simulink model "gm_hdl_model_fixed"  (R2024a)
settings: Solver=FixedStepDiscrete  StartTime=0.0  StopTime=SIM_TIME  RelTol=1e-3
undefined symbols (not defined in the file or in its folder): a, b, BUFFER_LEN, c, SAMPLING_FREQ, signal_1
libraries: hdlsllib x39, dspsigops x15, simulink_extras x4, simulink x2, dspsrcs4 x1, dsphdlxfrm2 x1
(part 1 of 3)
settings Model: SimulationMode=accelerator  Creator=Jan Rosa  LastModifiedBy=Jan Rosa
settings OptimizationCC: BlockReduction=off  ConditionallyExecuteInputs=off  DefaultParameterBehavior=Inlined  InheritOutputTypeSmallerThanSingle=on
settings DebuggingCC: SignalRangeChecking=warning  AlgebraicLoopMsg=error  SolverPrmCheckMsg=warning  InheritedTsInSrcMsg=none  SingleTaskRateTransMsg=error  UnderSpecifiedDataTypeMsg=warning  UnconnectedInputMsg=error  UnconnectedOutputMsg=error  UnconnectedLineMsg=error  ModelReferenceVersionMismatchMessage=warning  ModelReferenceIOMismatchMessage=warning  ModelReferenceNoExplicitFinalValueMsg=warning  StateNameClashWarn=warning
settings HardwareCC: ProdBitPerPointer=32  ProdBitPerSizeT=32  ProdBitPerPtrDiffT=32  ProdLargestAtomicFloat=None  ProdIntDivRoundTo=Undefined  ProdEndianess=Unspecified  ProdWordSize=32  ProdHWDeviceType=ASIC/FPGA->ASIC/FPGA  TargetBitPerPointer=64  TargetBitPerSizeT=64  TargetBitPerPtrDiffT=64  TargetLongLongMode=on  TargetIntDivRoundTo=Zero  TargetEndianess=LittleEndian  TargetWordSize=64  TargetHWDeviceType=Custom Processor->MATLAB Host Computer  ProdEqTarget=off
settings ModelReferenceCC: EnableRefExpFcnMdlSchedulingChecks=on  EnableParallelModelReferenceBuilds=on

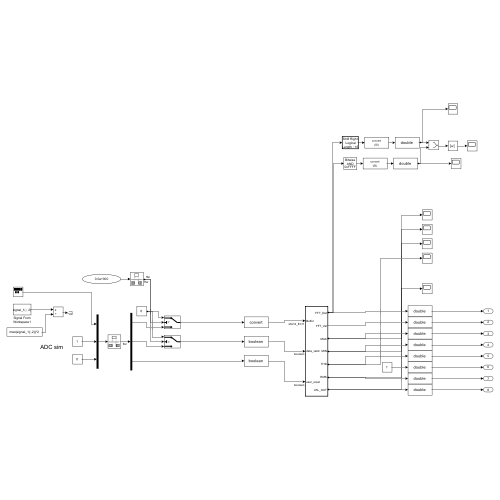
[thumbnail: Simulink's stored preview of the top-level diagram]
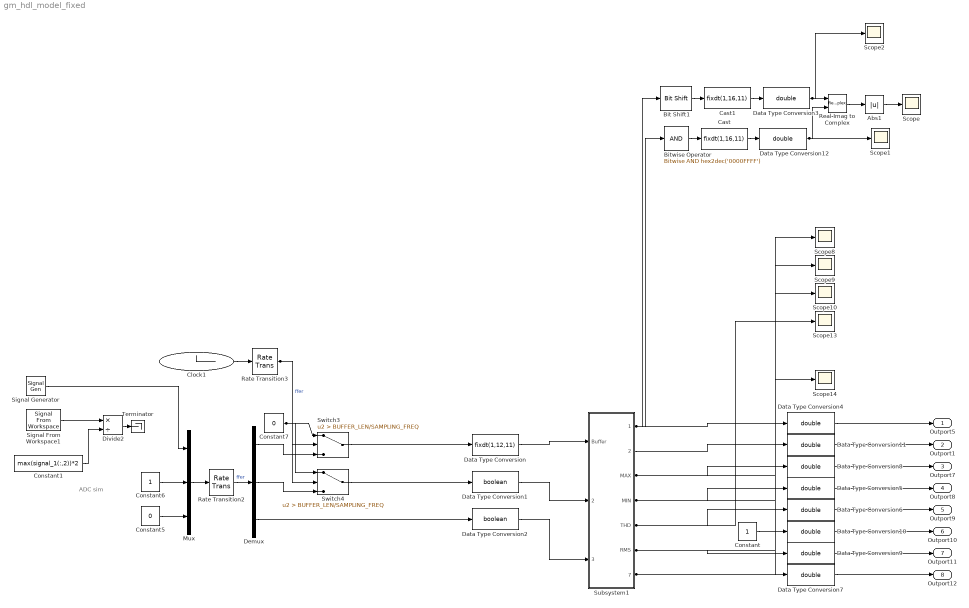
== system gm_hdl_model_fixed ==
  note: ADC sim
  Abs1 : Abs  SaturateOnIntegerOverflow=off
  Bit Shift1 : hdlsllib/Logic and Bit Operations/Bit Shift  mode=Shift Right Logical  N=16
  Bitwise Operator : simulink/Logic and Bit Operations/Bitwise Operator  logicop=AND  UseBitMask=on  BitMask=hex2dec('0000FFFF')  BitMaskRealWorld=Stored Integer
  Cast : DataTypeConversion  OutDataTypeStr=fixdt(1,16,11)  ConvertRealWorld=Stored Integer (SI)  SaturateOnIntegerOverflow=off  RndMeth=Floor
  Cast1 : DataTypeConversion  OutDataTypeStr=fixdt(1,16,11)  ConvertRealWorld=Stored Integer (SI)  SaturateOnIntegerOverflow=off  RndMeth=Floor
  Clock1 : Clock
  Constant : Constant
  Constant1 : Constant  Value=max(signal_1(:,2))*2
  Constant5 : Constant  Value=0
  Constant6 : Constant
  Constant7 : Constant  Value=0  SampleTime=1/SAMPLING_FREQ
  Data Type Conversion : DataTypeConversion  OutDataTypeStr=fixdt(1,12,11)  SaturateOnIntegerOverflow=off  RndMeth=Floor  LockScale=on
  Data Type Conversion1 : DataTypeConversion  OutDataTypeStr=boolean  SaturateOnIntegerOverflow=off  RndMeth=Floor  LockScale=on
  Data Type Conversion{3..12} (10 alike) : DataTypeConversion  OutDataTypeStr=double  SaturateOnIntegerOverflow=off  RndMeth=Floor
  Data Type Conversion2 : DataTypeConversion  OutDataTypeStr=boolean  SaturateOnIntegerOverflow=off  RndMeth=Floor  LockScale=on
  Demux : Demux  Outputs=3
  Divide2 : Product  Inputs=*/
  Mux : Mux  Inputs=3
  Rate Transition2 : RateTransition  Integrity=off  Deterministic=off  OutPortSampleTime=1/SAMPLING_FREQ
  Rate Transition3 : RateTransition  Integrity=off  Deterministic=off  OutPortSampleTime=1/SAMPLING_FREQ
  Real-Imag to Complex : RealImagToComplex
  Scope{,1..2,8..10,13..14} (8 alike) : Scope
  Signal Generator : SignalGenerator  WaveForm=square  Amplitude=0.49999  Frequency=SAMPLING_FREQ/(16*16)
  Signal From Workspace1 : dspsrcs4/Signal From Workspace  X=signal_1(:, 2)  Ts=signal_1(2, 1)  nsamps=1  OutputAfterFinalValue=Cyclic repetition  ignoreOrWarnInputAndFrameLengths=off  OutputFrames=off
  Subsystem1 : Subsystem  TreatAsAtomicUnit=on
  Switch3 : Switch  Criteria=u2 > Threshold  Threshold=BUFFER_LEN/SAMPLING_FREQ  SaturateOnIntegerOverflow=off  InputSameDT=off
  Switch4 : Switch  Criteria=u2 > Threshold  Threshold=BUFFER_LEN/SAMPLING_FREQ  SaturateOnIntegerOverflow=off  InputSameDT=off
  Terminator : Terminator
  Outport5 : Outport
  Outport1 : Outport  Port=2
  Outport7 : Outport  Port=3
  Outport8 : Outport  Port=4
  Outport9 : Outport  Port=5
  Outport10 : Outport  Port=6
  Outport11 : Outport  Port=7
  Outport12 : Outport  Port=8
  wires:
  Divide2/1 -> Terminator/1
  Constant/1 -> Data Type Conversion10/1
  Cast1/1 -> Data Type Conversion3/1
  Cast/1 -> Data Type Conversion12/1
  Data Type Conversion12/1 -> Real-Imag to Complex/2, Scope1/1
  Bitwise Operator/1 -> Cast/1
  Bit Shift1/1 -> Cast1/1
  Signal Generator/1 -> Mux/1
  Real-Imag to Complex/1 -> Abs1/1
  Subsystem1/2(FFT_Val) -> Data Type Conversion11/1
  Data Type Conversion3/1 -> Real-Imag to Complex/1, Scope2/1
  Data Type Conversion11/1 -> Outport1/1
  Data Type Conversion9/1 -> Outport11/1
  Data Type Conversion7/1 -> Outport12/1
  Data Type Conversion10/1 -> Outport10/1
  Data Type Conversion6/1 -> Outport9/1
  Data Type Conversion5/1 -> Outport8/1
  Data Type Conversion8/1 -> Outport7/1
  Data Type Conversion4/1 -> Outport5/1
  Data Type Conversion1/1 -> Subsystem1/2(data_valid)
  Data Type Conversion2/1 -> Subsystem1/3(user_reset)
  Data Type Conversion/1 -> Subsystem1/1(Buffer)
  Subsystem1/6(RMS) -> Scope8/1, Data Type Conversion9/1
  Constant1/1 -> Divide2/2
  Constant6/1 -> Mux/2
  Signal From Workspace1/1 -> Divide2/1
  Constant5/1 -> Mux/3
  Rate Transition2/1 -> Demux/1  "ffer"
  Abs1/1 -> Scope/1
  Subsystem1/4(MIN) -> Scope9/1, Data Type Conversion5/1
  Mux/1 -> Rate Transition2/1
  Demux/1 -> Switch3/3
  Switch3/1 -> Data Type Conversion/1
  Subsystem1/5(THD) -> Scope13/1, Data Type Conversion6/1
  Demux/3 -> Data Type Conversion2/1
  Clock1/1 -> Rate Transition3/1
  Demux/2 -> Switch4/3
  Subsystem1/3(MAX) -> Scope10/1, Data Type Conversion8/1
  Subsystem1/7(VAL_OUT) -> Scope14/1, Data Type Conversion7/1
  Rate Transition3/1 -> Switch3/2, Switch4/2  "ffer"
  Constant7/1 -> Switch3/1, Switch4/1
  Switch4/1 -> Data Type Conversion1/1
  Subsystem1/1(FFT_Dat) -> Bit Shift1/1, Bitwise Operator/1, Data Type Conversion4/1

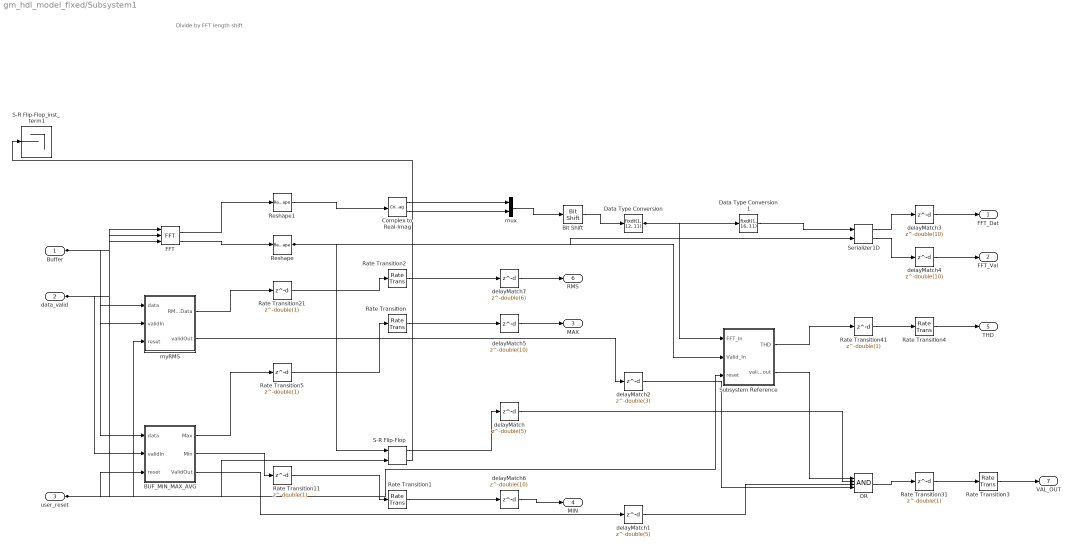
== system gm_hdl_model_fixed/Subsystem1 ==
  note: Divide by FFT length shift
  Buffer : Inport  OutDataTypeStr=fixdt(1, 12, 11)  PortDimensions=1  SampleTime=1e-08
  data_valid : Inport  Port=2  OutDataTypeStr=boolean  PortDimensions=1  SampleTime=1e-08
  user_reset : Inport  Port=3  OutDataTypeStr=boolean  PortDimensions=1  SampleTime=1e-08
  BUF_MIN_MAX_AVG : Subsystem
  Bit Shift : hdlsllib/Logic and Bit Operations/Bit Shift  mode=Shift Right Arithmetic  N=double(11)
  Complex to Real-Imag : ComplexToRealImag  SampleTime=1e-08
  Data Type Conversion : DataTypeConversion  OutDataTypeStr=fixdt(1, 12, 11)  SampleTime=1e-08  SaturateOnIntegerOverflow=off  RndMeth=Floor
  Data Type Conversion1 : DataTypeConversion  OutDataTypeStr=fixdt(1, 16, 11)  SampleTime=1e-08  SaturateOnIntegerOverflow=off  RndMeth=Floor
  FFT : dsphdlxfrm2/FFT  Architecture=Streaming Radix 2^2  FFTLengthSource=Property  FFTLength=BUFFER_LEN  FFTLengthMax=1024  ComplexMultiplication=Use 4 multipliers and 2 adders  BitReversedOutput=off  BitReversedInput=off  Normalize=off  SimulateUsing=Code generation  RoundingMethod=Floor  ResetInputPort=on  StartOutputPort=off  EndOutputPort=off
  OR : Logic  Inputs=4  AllPortsSameDT=off  OutDataTypeStr=boolean  SampleTime=1e-08
  Rate Transition : RateTransition  Integrity=off  Deterministic=off  InitialCondition="fi(0,0,16,16,\"hex\",\"0000\")"  OutPortSampleTimeOpt=Multiple of input port sample time  OutPortSampleTimeMultiple=1/2
  Rate Transition1 : RateTransition  Integrity=off  Deterministic=off  InitialCondition="fi(0,1,16,15,\"hex\",\"0000\")"  OutPortSampleTimeOpt=Multiple of input port sample time  OutPortSampleTimeMultiple=1/2
  Rate Transition{5,11,21,31,41} (5 alike) : Delay  DelayLength=double(1)  InitialCondition=0  SampleTime=1e-08
  Rate Transition2 : RateTransition  Integrity=off  Deterministic=off  InitialCondition="fi(0,0,16,7,\"hex\",\"0000\")"  OutPortSampleTimeOpt=Multiple of input port sample time  OutPortSampleTimeMultiple=1/2
  Rate Transition3 : RateTransition  Integrity=off  Deterministic=off  OutPortSampleTimeOpt=Multiple of input port sample time  OutPortSampleTimeMultiple=1/2
  Rate Transition4 : RateTransition  Integrity=off  Deterministic=off  InitialCondition="fi(0,1,18,10,\"hex\",\"00000\")"  OutPortSampleTimeOpt=Multiple of input port sample time  OutPortSampleTimeMultiple=1/2
  Reshape : Reshape
  Reshape1 : Reshape
  S-R Flip-Flop : simulink_extras/Flip Flops/S-R Flip-Flop  initial_condition=0
  S-R Flip-Flop_inst_term1 : Terminator
  Serializer1D : hdlsllib/HDL Operations/Serializer1D  Ratio=2  IdleCycles=0  validIn=on  startOut=off  validOut=on  inputDataDimensions=2  inputSampleTime=1e-08  inputSignalType=real
  Subsystem Reference : Subsystem
  delayMatch : Delay  DelayLength=double(5)  InitialCondition=0  SampleTime=1e-08
  delayMatch1 : Delay  DelayLength=double(5)  InitialCondition=0  SampleTime=1e-08
  delayMatch2 : Delay  DelayLength=double(3)  InitialCondition=0  SampleTime=1e-08
  delayMatch{3..6} (4 alike) : Delay  DelayLength=double(10)  InitialCondition=0  SampleTime=5e-09
  delayMatch7 : Delay  DelayLength=double(6)  InitialCondition=0  SampleTime=5e-09
  mux : Mux  Inputs=2
  myRMS : Subsystem
  FFT_Dat : Outport  SampleTime=5e-09
  FFT_Val : Outport  Port=2  SampleTime=5e-09
  MAX : Outport  Port=3  SampleTime=5e-09
  MIN : Outport  Port=4  SampleTime=5e-09
  THD : Outport  Port=5  SampleTime=5e-09
  RMS : Outport  Port=6  SampleTime=5e-09
  VAL_OUT : Outport  Port=7  SampleTime=5e-09
  wires:
  Buffer/1 -> BUF_MIN_MAX_AVG/1(data), myRMS/1(data), FFT/1
  data_valid/1 -> BUF_MIN_MAX_AVG/2(validIn), myRMS/2(validIn), FFT/2
  user_reset/1 -> myRMS/3(reset), BUF_MIN_MAX_AVG/3(reset), Subsystem Reference/3(reset), S-R Flip-Flop/2, FFT/3
  BUF_MIN_MAX_AVG/1(Max) -> Rate Transition5/1
  BUF_MIN_MAX_AVG/2(Min) -> Rate Transition11/1
  delayMatch1/1 -> OR/3
  Data Type Conversion/1 -> Subsystem Reference/1(FFT_In), Data Type Conversion1/1
  FFT/1 -> Reshape1/1
  FFT/2 -> Reshape/1
  Reshape/1 -> Subsystem Reference/2(Valid_In), Serializer1D/2, S-R Flip-Flop/1
  delayMatch3/1 -> FFT_Dat/1
  Subsystem Reference/1(THD) -> Rate Transition41/1
  Subsystem Reference/2(valid_out) -> OR/1
  myRMS/1(RMS_Data) -> Rate Transition21/1
  delayMatch2/1 -> OR/4
  delayMatch5/1 -> MAX/1
  delayMatch6/1 -> MIN/1
  delayMatch7/1 -> RMS/1
  Rate Transition3/1 -> VAL_OUT/1
  Rate Transition4/1 -> THD/1
  delayMatch4/1 -> FFT_Val/1
  delayMatch/1 -> OR/2
  Rate Transition5/1 -> Rate Transition/1
  Rate Transition11/1 -> Rate Transition1/1
  Rate Transition21/1 -> Rate Transition2/1
  Rate Transition31/1 -> Rate Transition3/1
  Rate Transition41/1 -> Rate Transition4/1
  S-R Flip-Flop/2 -> S-R Flip-Flop_inst_term1/1
  Reshape1/1 -> Complex to Real-Imag/1
  Complex to Real-Imag/1 -> mux/1
  Complex to Real-Imag/2 -> mux/2
  mux/1 -> Bit Shift/1
  Bit Shift/1 -> Data Type Conversion/1
  Data Type Conversion1/1 -> Serializer1D/1
  OR/1 -> Rate Transition31/1
  S-R Flip-Flop/1 -> delayMatch/1
  BUF_MIN_MAX_AVG/3(ValidOut) -> delayMatch1/1
  myRMS/2(validOut) -> delayMatch2/1
  Serializer1D/1 -> delayMatch3/1
  Serializer1D/2 -> delayMatch4/1
  Rate Transition/1 -> delayMatch5/1
  Rate Transition1/1 -> delayMatch6/1
  Rate Transition2/1 -> delayMatch7/1

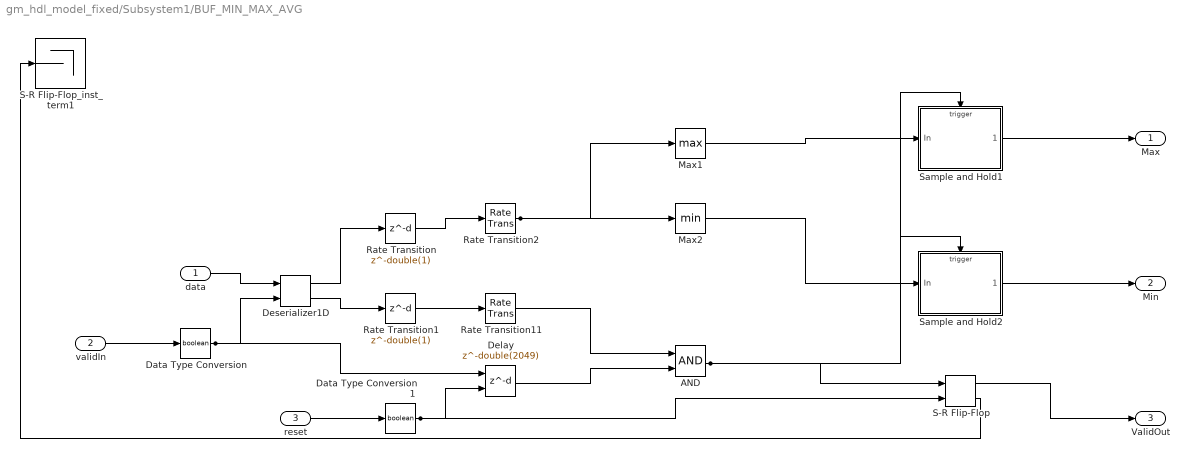
== system gm_hdl_model_fixed/Subsystem1/BUF_MIN_MAX_AVG ==
  data : Inport  OutDataTypeStr=fixdt(1, 12, 11)  PortDimensions=1  SampleTime=1e-08
  validIn : Inport  Port=2  OutDataTypeStr=boolean  PortDimensions=1  SampleTime=1e-08
  reset : Inport  Port=3  OutDataTypeStr=boolean  PortDimensions=1  SampleTime=1e-08
  AND : Logic  AllPortsSameDT=off  OutDataTypeStr=boolean  SampleTime=1e-08
  Data Type Conversion : DataTypeConversion  OutDataTypeStr=boolean
  Data Type Conversion1 : DataTypeConversion  OutDataTypeStr=boolean
  Delay : Delay  DelayLength=double(2049)  InitialCondition=0  ExternalReset=Level
      settings: InputPortMap=u0,r5
  Deserializer1D : hdlsllib/HDL Operations/Deserializer1D  Ratio=2048  IdleCycles=0  InitialCondition=0  startIn=off  validIn=on  validOut=on  inputDataDimensions=1  inputSampleTime=1e-08  inputSignalType=real
  Max1 : MinMax  Function=max  OutDataTypeStr=fixdt(0,16,16)
  Max2 : MinMax  OutDataTypeStr=fixdt(1,16,15)
  Rate Transition : Delay  DelayLength=double(1)  InitialCondition=0  SampleTime=2.048e-05
  Rate Transition1 : Delay  DelayLength=double(1)  InitialCondition=0  SampleTime=2.048e-05
  Rate Transition11 : RateTransition  Integrity=off  Deterministic=off  OutPortSampleTimeOpt=Multiple of input port sample time  OutPortSampleTimeMultiple=1/2048
  Rate Transition2 : RateTransition  Integrity=off  Deterministic=off  InitialCondition="fi(0,1,12,11,\"hex\",\"000\")"  OutPortSampleTimeOpt=Multiple of input port sample time  OutPortSampleTimeMultiple=1/2048
  S-R Flip-Flop : simulink_extras/Flip Flops/S-R Flip-Flop  initial_condition=0
  S-R Flip-Flop_inst_term1 : Terminator
  Sample and Hold1 : Subsystem  mask(Sample and Hold){trig=Rising edge, initCond=double(0), latchinput=off}
      mask prompts: trig "dsp:DSPSignalOperationsBlockDialog:TriggerType_MP"; initCond "dsp:DSPSignalOperationsBlockDialog:InitialCondition_MP"; latchinput "dsp:DSPSignalOperationsBlockDialog:LatchInput_MP"
      mask help: dsp:DSPSignalOperationsBlockDialog:SampleAndHold_MaskDesc
      mask init:
      | initCond = double(0);
      | latchinput = double(0);
      | s = 'rising';
      | trig = double(1);
      mask Help: eval('blocksethelp');
      mask TypeOptions trig: dsp:DSPSignalOperationsBlockDialog:RisingEdge_MP | dsp:DSPSignalOperationsBlockDialog:FallingEdge_MP | dsp:DSPSignalOperationsBlockDialog:EitherEdge_MP
      mask Display: disp('S/H')
  Sample and Hold2 : Subsystem  mask(Sample and Hold){trig=Rising edge, initCond=double(0), latchinput=off}
      mask prompts: trig "dsp:DSPSignalOperationsBlockDialog:TriggerType_MP"; initCond "dsp:DSPSignalOperationsBlockDialog:InitialCondition_MP"; latchinput "dsp:DSPSignalOperationsBlockDialog:LatchInput_MP"
      mask help: dsp:DSPSignalOperationsBlockDialog:SampleAndHold_MaskDesc
      mask init:
      | initCond = double(0);
      | latchinput = double(0);
      | s = 'rising';
      | trig = double(1);
      mask Help: eval('blocksethelp');
      mask TypeOptions trig: dsp:DSPSignalOperationsBlockDialog:RisingEdge_MP | dsp:DSPSignalOperationsBlockDialog:FallingEdge_MP | dsp:DSPSignalOperationsBlockDialog:EitherEdge_MP
      mask Display: disp('S/H')
  Max : Outport  SampleTime=1e-08
  Min : Outport  Port=2  SampleTime=1e-08
  ValidOut : Outport  Port=3  SampleTime=1e-08
  wires:
  data/1 -> Deserializer1D/1
  validIn/1 -> Data Type Conversion/1
  reset/1 -> Data Type Conversion1/1
  Delay/1 -> AND/2
  S-R Flip-Flop/1 -> ValidOut/1
  Sample and Hold1/1(" ") -> Max/1
  Sample and Hold2/1(" ") -> Min/1
  Deserializer1D/2 -> Rate Transition1/1
  Data Type Conversion1/1 -> Delay/2, S-R Flip-Flop/2
  Max2/1 -> Sample and Hold2/1(In)
  Max1/1 -> Sample and Hold1/1(In)
  Rate Transition1/1 -> Rate Transition11/1
  Rate Transition/1 -> Rate Transition2/1
  Rate Transition11/1 -> AND/1
  Rate Transition2/1 -> Max2/1, Max1/1
  Data Type Conversion/1 -> Deserializer1D/2, Delay/1
  AND/1 -> Sample and Hold1/Trigger, Sample and Hold2/Trigger, S-R Flip-Flop/1
  S-R Flip-Flop/2 -> S-R Flip-Flop_inst_term1/1
  Deserializer1D/1 -> Rate Transition/1

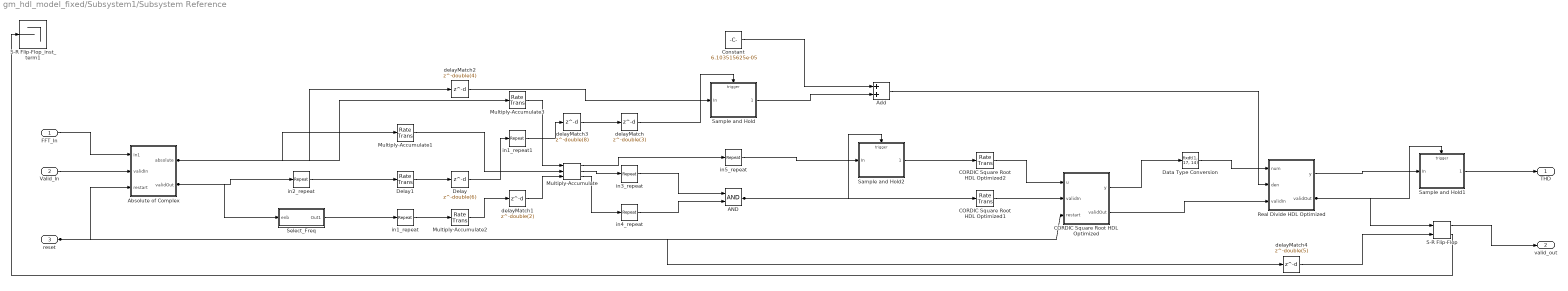
== system gm_hdl_model_fixed/Subsystem1/Subsystem Reference ==
  FFT_In : Inport  OutDataTypeStr=fixdt(1, 12, 11)  PortDimensions=[2]  SampleTime=1e-08
  Valid_In : Inport  Port=2  OutDataTypeStr=boolean  PortDimensions=1  SampleTime=1e-08
  reset : Inport  Port=3  OutDataTypeStr=boolean  PortDimensions=1  SampleTime=1e-08
  AND : Logic  AllPortsSameDT=off  OutDataTypeStr=boolean  SampleTime=5e-09
  Absolute of Complex : Subsystem
  Add : Sum  OutDataTypeStr=fixdt(1, 17, 14)  AccumDataTypeStr=fixdt(1, 17, 14)  SampleTime=5e-09
  CORDIC Square Root HDL Optimized : Subsystem  mask(CORDIC Square Root HDL Optimized){autoMaximumShiftVal=on, maximumShiftValue=double(10), nIterPerReg=double(1)}
      mask prompts: autoMaximumShiftVal "fixed:emblib:AutoCORDICMaxShiftValue"; maximumShiftValue "fixed:emblib:CORDICMaxShiftValue"; nIterPerReg "fixed:emblib:NumberOfIterationsPerReg"
      mask help: fixed:emblib:CORDICSquareRootHDLFullDescription
      mask Help: eval('embblk.embhelp(gcb)')
      mask Callback autoMaximumShiftVal:
      | autoMaxShiftVal = get_param(gcb,'autoMaximumShiftVal');
      | if strcmp(autoMaxShiftVal,'on')
      |     set_param(gcb,'MaskVisibilities',{'on','off','on'});
      | else
      |     set_param(gcb,'MaskVisibilities',{'on','on','on'});
      | end
      mask Display: disp('CORDIC Square Root\nHDL Optimized')
  CORDIC Square Root HDL Optimized1 : RateTransition  OutPortSampleTimeOpt=Multiple of input port sample time  OutPortSampleTimeMultiple=2
  CORDIC Square Root HDL Optimized2 : RateTransition  OutPortSampleTimeOpt=Multiple of input port sample time  OutPortSampleTimeMultiple=2
  Constant : Constant  Value=6.103515625e-05  OutDataTypeStr=fixdt(1, 16, 14)  SampleTime=5e-09
  Data Type Conversion : DataTypeConversion  OutDataTypeStr=fixdt(1, 17, 14)  SampleTime=1e-08  SaturateOnIntegerOverflow=off  RndMeth=Floor
  Delay : Delay  DelayLength=double(6)  InitialCondition=0  SampleTime=1e-08
  Delay1 : RateTransition  OutPortSampleTimeOpt=Multiple of input port sample time  OutPortSampleTimeMultiple=2
  Multiply-Accumulate : hdlsllib/HDL Operations/Multiply-Accumulate  opMode=Streaming - using Number of Samples  initValueSetting=Dialog  initValue=0  initValueSetting2=Dialog  initValue2=0  initValueSetting3=Dialog  initValue3=0  num_samples=1015  RndMeth2=Floor  RndMeth3=Floor  datatype2=Inherit: Inherit via back propagation  datatype3=fixdt(1, 22, 20)  validOut=on  endInandOut=on  startOut=on  countOut=off  dim=-1  DoSatur=off  parallel=off
  Multiply-Accumulate1 : RateTransition  OutPortSampleTimeOpt=Multiple of input port sample time  OutPortSampleTimeMultiple=2
  Multiply-Accumulate2 : RateTransition  OutPortSampleTimeOpt=Multiple of input port sample time  OutPortSampleTimeMultiple=2
  Multiply-Accumulate3 : RateTransition  OutPortSampleTimeOpt=Multiple of input port sample time  OutPortSampleTimeMultiple=2
  Real Divide HDL Optimized : Subsystem  mask(Real Divide HDL Optimized){OutputType=fixdt(1,18,10)}
      mask prompts: OutputType "fixed:emblib:OutputPrototype"
      mask help: fixed:emblib:RealDivideFullDescription
      mask Help: eval('embblk.embhelp(gcb)')
      mask Display:
      | text(0.5,0.6,'den ~= 0','texmode','on','HorizontalAlignment','center')
      | text(0.5,0.4,'y = num/den','texmode','on','HorizontalAlignment','center')
  S-R Flip-Flop : simulink_extras/Flip Flops/S-R Flip-Flop  initial_condition=0
  S-R Flip-Flop_inst_term1 : Terminator
  Sample and Hold : Subsystem  mask(Sample and Hold){trig=Rising edge, initCond=double(0), latchinput=off}
      mask prompts: trig "dsp:DSPSignalOperationsBlockDialog:TriggerType_MP"; initCond "dsp:DSPSignalOperationsBlockDialog:InitialCondition_MP"; latchinput "dsp:DSPSignalOperationsBlockDialog:LatchInput_MP"
      mask help: dsp:DSPSignalOperationsBlockDialog:SampleAndHold_MaskDesc
      mask init:
      | initCond = double(0);
      | latchinput = double(0);
      | s = 'rising';
      | trig = double(1);
      mask Help: eval('blocksethelp');
      mask TypeOptions trig: dsp:DSPSignalOperationsBlockDialog:RisingEdge_MP | dsp:DSPSignalOperationsBlockDialog:FallingEdge_MP | dsp:DSPSignalOperationsBlockDialog:EitherEdge_MP
      mask Display: disp('S/H')
  Sample and Hold1 : Subsystem  mask(Sample and Hold){trig=Rising edge, initCond=double(0), latchinput=off}
      mask prompts: trig "dsp:DSPSignalOperationsBlockDialog:TriggerType_MP"; initCond "dsp:DSPSignalOperationsBlockDialog:InitialCondition_MP"; latchinput "dsp:DSPSignalOperationsBlockDialog:LatchInput_MP"
      mask help: dsp:DSPSignalOperationsBlockDialog:SampleAndHold_MaskDesc
      mask init:
      | initCond = double(0);
      | latchinput = double(0);
      | s = 'rising';
      | trig = double(1);
      mask Help: eval('blocksethelp');
      mask TypeOptions trig: dsp:DSPSignalOperationsBlockDialog:RisingEdge_MP | dsp:DSPSignalOperationsBlockDialog:FallingEdge_MP | dsp:DSPSignalOperationsBlockDialog:EitherEdge_MP
      mask Display: disp('S/H')
  Sample and Hold2 : Subsystem  mask(Sample and Hold){trig=Rising edge, initCond=double(0), latchinput=off}
      mask prompts: trig "dsp:DSPSignalOperationsBlockDialog:TriggerType_MP"; initCond "dsp:DSPSignalOperationsBlockDialog:InitialCondition_MP"; latchinput "dsp:DSPSignalOperationsBlockDialog:LatchInput_MP"
      mask help: dsp:DSPSignalOperationsBlockDialog:SampleAndHold_MaskDesc
      mask init:
      | initCond = double(0);
      | latchinput = double(0);
      | s = 'rising';
      | trig = double(1);
      mask Help: eval('blocksethelp');
      mask TypeOptions trig: dsp:DSPSignalOperationsBlockDialog:RisingEdge_MP | dsp:DSPSignalOperationsBlockDialog:FallingEdge_MP | dsp:DSPSignalOperationsBlockDialog:EitherEdge_MP
      mask Display: disp('S/H')
  Select_Freq : Subsystem
  delayMatch : Delay  DelayLength=double(3)  InitialCondition=0  SampleTime=5e-09
  delayMatch1 : Delay  DelayLength=double(2)  InitialCondition=0  SampleTime=1e-08
  delayMatch2 : Delay  DelayLength=double(4)  InitialCondition=0  SampleTime=5e-09
  delayMatch3 : Delay  DelayLength=double(8)  InitialCondition=0  SampleTime=5e-09
  delayMatch4 : Delay  DelayLength=double(5)  InitialCondition=0  SampleTime=1e-08
  in1_repeat : dspsigops/Repeat  FactorSource=Dialog parameter  N=double(2)  Nmax=16  RateOptions=Allow multirate processing  ic=0  mode=Unused parameter value
  in1_repeat1 : dspsigops/Repeat  FactorSource=Dialog parameter  N=double(2)  Nmax=16  RateOptions=Allow multirate processing  ic=0  mode=Unused parameter value
  in2_repeat : dspsigops/Repeat  FactorSource=Dialog parameter  N=double(2)  Nmax=16  RateOptions=Allow multirate processing  ic=0  mode=Unused parameter value
  in3_repeat : dspsigops/Repeat  FactorSource=Dialog parameter  N=double(2)  Nmax=16  RateOptions=Allow multirate processing  ic=0  mode=Unused parameter value
  in4_repeat : dspsigops/Repeat  FactorSource=Dialog parameter  N=double(2)  Nmax=16  RateOptions=Allow multirate processing  ic=0  mode=Unused parameter value
  in5_repeat : dspsigops/Repeat  FactorSource=Dialog parameter  N=double(2)  Nmax=16  RateOptions=Allow multirate processing  ic=0  mode=Unused parameter value
  THD : Outport  SampleTime=1e-08
  valid_out : Outport  Port=2  SampleTime=1e-08
  wires:
  FFT_In/1 -> Absolute of Complex/1(In1)
  Valid_In/1 -> Absolute of Complex/2(validIn)
  delayMatch4/1 -> S-R Flip-Flop/2
  CORDIC Square Root HDL Optimized1/1 -> CORDIC Square Root HDL Optimized/2(validIn)
  Absolute of Complex/2(validOut) -> Select_Freq/1(enb), in2_repeat/1
  CORDIC Square Root HDL Optimized/1(y) -> Data Type Conversion/1
  CORDIC Square Root HDL Optimized/2(validOut) -> Real Divide HDL Optimized/3(validIn)
  Data Type Conversion/1 -> Real Divide HDL Optimized/1(num)
  Multiply-Accumulate/1 -> in5_repeat/1
  Multiply-Accumulate/2 -> in3_repeat/1
  Multiply-Accumulate/3 -> in4_repeat/1
  Real Divide HDL Optimized/1(y) -> Sample and Hold1/1(In)
  Real Divide HDL Optimized/2(validOut) -> Sample and Hold1/Trigger, S-R Flip-Flop/1
  S-R Flip-Flop/1 -> valid_out/1
  Sample and Hold1/1(" ") -> THD/1
  CORDIC Square Root HDL Optimized2/1 -> CORDIC Square Root HDL Optimized/1(u)
  Select_Freq/1(Out1) -> in1_repeat/1
  S-R Flip-Flop/2 -> S-R Flip-Flop_inst_term1/1
  Add/1 -> Real Divide HDL Optimized/2(den)
  delayMatch2/1 -> Sample and Hold/1(In)
  Delay1/1 -> Delay/1
  Multiply-Accumulate1/1 -> Multiply-Accumulate/2
  delayMatch1/1 -> Multiply-Accumulate/3
  Delay/1 -> in1_repeat1/1
  Multiply-Accumulate3/1 -> Multiply-Accumulate/1
  in1_repeat/1 -> Multiply-Accumulate2/1
  in2_repeat/1 -> Delay1/1
  Constant/1 -> Add/1
  delayMatch3/1 -> delayMatch/1
  in3_repeat/1 -> AND/1
  in4_repeat/1 -> AND/2
  in5_repeat/1 -> Sample and Hold2/1(In)
  AND/1 -> CORDIC Square Root HDL Optimized1/1, Sample and Hold2/Trigger
  Sample and Hold2/1(" ") -> CORDIC Square Root HDL Optimized2/1
  Multiply-Accumulate2/1 -> delayMatch1/1
  Absolute of Complex/1(absolute) -> delayMatch2/1, Multiply-Accumulate3/1, Multiply-Accumulate1/1
  in1_repeat1/1 -> delayMatch3/1
  reset/1 -> delayMatch4/1, Absolute of Complex/3(restart), CORDIC Square Root HDL Optimized/3(restart)
  delayMatch/1 -> Sample and Hold/Trigger
  Sample and Hold/1(" ") -> Add/2

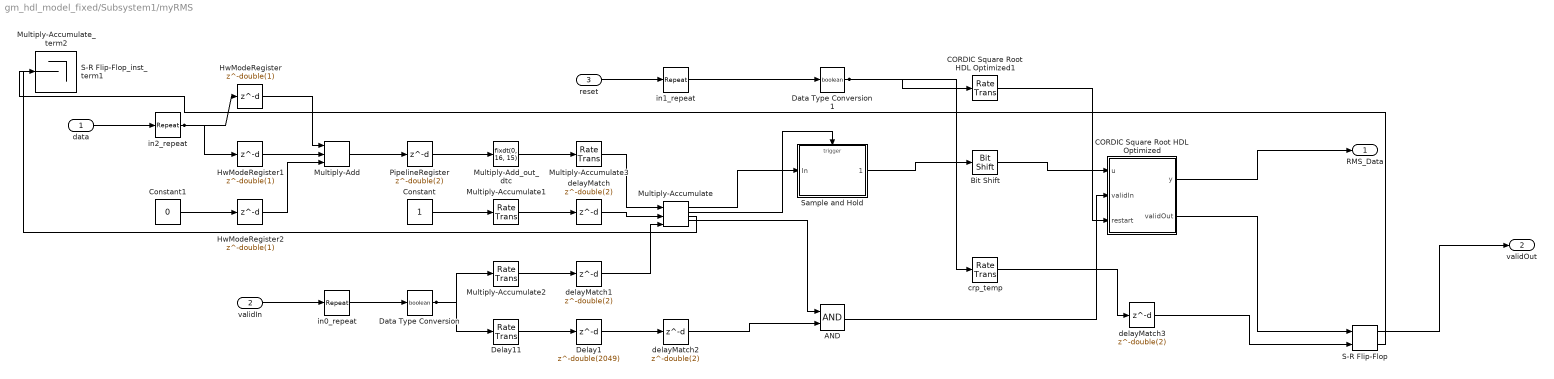
== system gm_hdl_model_fixed/Subsystem1/myRMS ==
  data : Inport  OutDataTypeStr=fixdt(1, 12, 11)  PortDimensions=1  SampleTime=1e-08
  validIn : Inport  Port=2  OutDataTypeStr=boolean  PortDimensions=1  SampleTime=1e-08
  reset : Inport  Port=3  OutDataTypeStr=boolean  PortDimensions=1  SampleTime=1e-08
  AND : Logic  AllPortsSameDT=off  OutDataTypeStr=boolean  SampleTime=1e-08
  Bit Shift : hdlsllib/Logic and Bit Operations/Bit Shift  mode=Shift Right Arithmetic  N=double(11)
  CORDIC Square Root HDL Optimized : Subsystem  mask(CORDIC Square Root HDL Optimized){autoMaximumShiftVal=on, maximumShiftValue=double(10), nIterPerReg=double(1)}
      mask prompts: autoMaximumShiftVal "fixed:emblib:AutoCORDICMaxShiftValue"; maximumShiftValue "fixed:emblib:CORDICMaxShiftValue"; nIterPerReg "fixed:emblib:NumberOfIterationsPerReg"
      mask help: fixed:emblib:CORDICSquareRootHDLFullDescription
      mask Help: eval('embblk.embhelp(gcb)')
      mask Callback autoMaximumShiftVal:
      | autoMaxShiftVal = get_param(gcb,'autoMaximumShiftVal');
      | if strcmp(autoMaxShiftVal,'on')
      |     set_param(gcb,'MaskVisibilities',{'on','off','on'});
      | else
      |     set_param(gcb,'MaskVisibilities',{'on','on','on'});
      | end
      mask Display: disp('CORDIC Square Root\nHDL Optimized')
  CORDIC Square Root HDL Optimized1 : RateTransition  OutPortSampleTimeOpt=Multiple of input port sample time  OutPortSampleTimeMultiple=2
  Constant : Constant  OutDataTypeStr=fixdt(0, 16, 15)  SampleTime=5e-09
  Constant1 : Constant  Value=0  OutDataTypeStr=fixdt(1, 12, 11)  SampleTime=5e-09
  Data Type Conversion : DataTypeConversion  OutDataTypeStr=boolean
  Data Type Conversion1 : DataTypeConversion  OutDataTypeStr=boolean
  Delay1 : Delay  DelayLength=double(2049)  InitialCondition=0  SampleTime=1e-08
  Delay11 : RateTransition  OutPortSampleTimeOpt=Multiple of input port sample time  OutPortSampleTimeMultiple=2
  HwModeRegister : Delay  DelayLength=double(1)  InitialCondition=0  SampleTime=5e-09
  HwModeRegister1 : Delay  DelayLength=double(1)  InitialCondition=0  SampleTime=5e-09
  HwModeRegister2 : Delay  DelayLength=double(1)  InitialCondition=0  SampleTime=5e-09
  Multiply-Accumulate : hdlsllib/HDL Operations/Multiply-Accumulate  opMode=Streaming - using Number of Samples  initValueSetting=Dialog  initValue=0  initValueSetting2=Dialog  initValue2=0  initValueSetting3=Dialog  initValue3=0  num_samples=2048  RndMeth2=Floor  RndMeth3=Floor  datatype2=Inherit: Inherit via back propagation  datatype3=fixdt(0, 16, 7)  validOut=on  endInandOut=on  startOut=on  countOut=on  dim=-1  DoSatur=off  parallel=off
  Multiply-Accumulate1 : RateTransition  OutPortSampleTimeOpt=Multiple of input port sample time  OutPortSampleTimeMultiple=2
  Multiply-Accumulate2 : RateTransition  OutPortSampleTimeOpt=Multiple of input port sample time  OutPortSampleTimeMultiple=2
  Multiply-Accumulate3 : RateTransition  OutPortSampleTimeOpt=Multiple of input port sample time  OutPortSampleTimeMultiple=2
  Multiply-Accumulate_term2 : Terminator
  Multiply-Add : hdlsllib/HDL Operations/Multiply-Add  Function=c+(a.*b)  datatype=fixdt(1, 25, 22)  DoSatur=off  FMA=off
  Multiply-Add_out_dtc : DataTypeConversion  OutDataTypeStr=fixdt(0, 16, 15)  SampleTime=5e-09  SaturateOnIntegerOverflow=off  RndMeth=Floor
  PipelineRegister : Delay  DelayLength=double(2)  InitialCondition=0  SampleTime=5e-09
  S-R Flip-Flop : simulink_extras/Flip Flops/S-R Flip-Flop  initial_condition=0
  S-R Flip-Flop_inst_term1 : Terminator
  Sample and Hold : Subsystem  mask(Sample and Hold){trig=Rising edge, initCond=double(0), latchinput=off}
      mask prompts: trig "dsp:DSPSignalOperationsBlockDialog:TriggerType_MP"; initCond "dsp:DSPSignalOperationsBlockDialog:InitialCondition_MP"; latchinput "dsp:DSPSignalOperationsBlockDialog:LatchInput_MP"
      mask help: dsp:DSPSignalOperationsBlockDialog:SampleAndHold_MaskDesc
      mask init:
      | initCond = double(0);
      | latchinput = double(0);
      | s = 'rising';
      | trig = double(1);
      mask Help: eval('blocksethelp');
      mask TypeOptions trig: dsp:DSPSignalOperationsBlockDialog:RisingEdge_MP | dsp:DSPSignalOperationsBlockDialog:FallingEdge_MP | dsp:DSPSignalOperationsBlockDialog:EitherEdge_MP
      mask Display: disp('S/H')
  crp_temp : RateTransition  OutPortSampleTimeOpt=Multiple of input port sample time  OutPortSampleTimeMultiple=2
  delayMatch{,1..3} (4 alike) : Delay  DelayLength=double(2)  InitialCondition=0  SampleTime=1e-08
  in0_repeat : dspsigops/Repeat  FactorSource=Dialog parameter  N=double(2)  Nmax=16  RateOptions=Allow multirate processing  ic=0  mode=Unused parameter value
  in1_repeat : dspsigops/Repeat  FactorSource=Dialog parameter  N=double(2)  Nmax=16  RateOptions=Allow multirate processing  ic=0  mode=Unused parameter value
  in2_repeat : dspsigops/Repeat  FactorSource=Dialog parameter  N=double(2)  Nmax=16  RateOptions=Allow multirate processing  ic=0  mode=Unused parameter value
  RMS_Data : Outport  SampleTime=1e-08
  validOut : Outport  Port=2  SampleTime=1e-08
  wires:
  data/1 -> in2_repeat/1
  validIn/1 -> in0_repeat/1
  reset/1 -> in1_repeat/1
  AND/1 -> CORDIC Square Root HDL Optimized/2(validIn)
  Bit Shift/1 -> CORDIC Square Root HDL Optimized/1(u)
  CORDIC Square Root HDL Optimized/1(y) -> RMS_Data/1
  CORDIC Square Root HDL Optimized/2(validOut) -> S-R Flip-Flop/1
  Multiply-Accumulate/1 -> Sample and Hold/1(In)
  Multiply-Accumulate/2 -> Sample and Hold/Trigger
  Multiply-Accumulate/3 -> Multiply-Accumulate_term2/1
  Multiply-Accumulate/4 -> AND/1
  S-R Flip-Flop/1 -> validOut/1
  Sample and Hold/1(" ") -> Bit Shift/1
  S-R Flip-Flop/2 -> S-R Flip-Flop_inst_term1/1
  Delay11/1 -> Delay1/1
  delayMatch/1 -> Multiply-Accumulate/2
  delayMatch1/1 -> Multiply-Accumulate/3
  delayMatch2/1 -> AND/2
  CORDIC Square Root HDL Optimized1/1 -> CORDIC Square Root HDL Optimized/3(restart)
  delayMatch3/1 -> S-R Flip-Flop/2
  Multiply-Accumulate3/1 -> Multiply-Accumulate/1
  in0_repeat/1 -> Data Type Conversion/1
  in1_repeat/1 -> Data Type Conversion1/1
  in2_repeat/1 -> HwModeRegister/1, HwModeRegister1/1
  Constant/1 -> Multiply-Accumulate1/1
  Data Type Conversion/1 -> Delay11/1, Multiply-Accumulate2/1
  Data Type Conversion1/1 -> crp_temp/1, CORDIC Square Root HDL Optimized1/1
  Multiply-Add_out_dtc/1 -> Multiply-Accumulate3/1
  Multiply-Accumulate1/1 -> delayMatch/1
  Multiply-Accumulate2/1 -> delayMatch1/1
  Delay1/1 -> delayMatch2/1
  crp_temp/1 -> delayMatch3/1
  Constant1/1 -> HwModeRegister2/1
  PipelineRegister/1 -> Multiply-Add_out_dtc/1
  Multiply-Add/1 -> PipelineRegister/1
  HwModeRegister/1 -> Multiply-Add/1
  HwModeRegister1/1 -> Multiply-Add/2
  HwModeRegister2/1 -> Multiply-Add/3

== system gm_hdl_model_fixed/Subsystem1/BUF_MIN_MAX_AVG/Sample and Hold1 ==
  In : Inport  OutDataTypeStr=fixdt(0, 16, 16)
  Trigger : TriggerPort  VariantControl=(inherit)  OutDataTypeStr=boolean
  " " : Outport  InitialOutput=0
  wires:
  In/1 -> " "/1

== system gm_hdl_model_fixed/Subsystem1/BUF_MIN_MAX_AVG/Sample and Hold2 ==
  In : Inport  OutDataTypeStr=fixdt(1, 16, 15)
  Trigger : TriggerPort  VariantControl=(inherit)  OutDataTypeStr=boolean
  " " : Outport  InitialOutput=0
  wires:
  In/1 -> " "/1

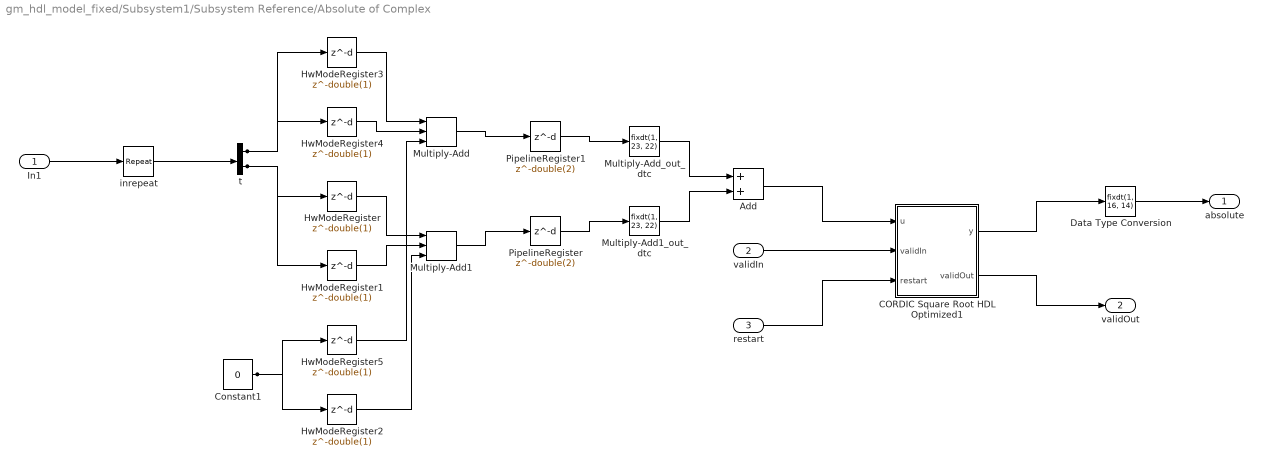
== system gm_hdl_model_fixed/Subsystem1/Subsystem Reference/Absolute of Complex ==
  In1 : Inport  OutDataTypeStr=fixdt(1, 12, 11)  PortDimensions=[2]  SampleTime=1e-08
  validIn : Inport  Port=2  OutDataTypeStr=boolean  PortDimensions=1  SampleTime=1e-08
  restart : Inport  Port=3  OutDataTypeStr=boolean  PortDimensions=1  SampleTime=1e-08
  Add : Sum  OutDataTypeStr=fixdt(1, 24, 22)  AccumDataTypeStr=fixdt(1, 24, 22)  SampleTime=5e-09
  CORDIC Square Root HDL Optimized1 : Subsystem  mask(CORDIC Square Root HDL Optimized){autoMaximumShiftVal=on, maximumShiftValue=double(10), nIterPerReg=double(1)}
      mask prompts: autoMaximumShiftVal "fixed:emblib:AutoCORDICMaxShiftValue"; maximumShiftValue "fixed:emblib:CORDICMaxShiftValue"; nIterPerReg "fixed:emblib:NumberOfIterationsPerReg"
      mask help: fixed:emblib:CORDICSquareRootHDLFullDescription
      mask Help: eval('embblk.embhelp(gcb)')
      mask Callback autoMaximumShiftVal:
      | autoMaxShiftVal = get_param(gcb,'autoMaximumShiftVal');
      | if strcmp(autoMaxShiftVal,'on')
      |     set_param(gcb,'MaskVisibilities',{'on','off','on'});
      | else
      |     set_param(gcb,'MaskVisibilities',{'on','on','on'});
      | end
      mask Display: disp('CORDIC Square Root\nHDL Optimized')
  Constant1 : Constant  Value=0  OutDataTypeStr=fixdt(1, 12, 11)  SampleTime=5e-09
  Data Type Conversion : DataTypeConversion  OutDataTypeStr=fixdt(1, 16, 14)  SampleTime=5e-09  SaturateOnIntegerOverflow=off  RndMeth=Floor
  HwModeRegister{,1..5} (6 alike) : Delay  DelayLength=double(1)  InitialCondition=0  SampleTime=5e-09
  Multiply-Add : hdlsllib/HDL Operations/Multiply-Add  Function=c+(a.*b)  datatype=fixdt(1, 25, 22)  DoSatur=off  FMA=off
  Multiply-Add1 : hdlsllib/HDL Operations/Multiply-Add  Function=c+(a.*b)  datatype=fixdt(1, 25, 22)  DoSatur=off  FMA=off
  Multiply-Add1_out_dtc : DataTypeConversion  OutDataTypeStr=fixdt(1, 23, 22)  SampleTime=5e-09  SaturateOnIntegerOverflow=off  RndMeth=Floor
  Multiply-Add_out_dtc : DataTypeConversion  OutDataTypeStr=fixdt(1, 23, 22)  SampleTime=5e-09  SaturateOnIntegerOverflow=off  RndMeth=Floor
  PipelineRegister : Delay  DelayLength=double(2)  InitialCondition=0  SampleTime=5e-09
  PipelineRegister1 : Delay  DelayLength=double(2)  InitialCondition=0  SampleTime=5e-09
  inrepeat : dspsigops/Repeat  FactorSource=Dialog parameter  N=double(2)  Nmax=16  RateOptions=Allow multirate processing  ic=0  mode=Unused parameter value
  t : Demux  Outputs=2
  absolute : Outport  SampleTime=5e-09
  validOut : Outport  Port=2  SampleTime=1e-08
  wires:
  In1/1 -> inrepeat/1
  validIn/1 -> CORDIC Square Root HDL Optimized1/2(validIn)
  restart/1 -> CORDIC Square Root HDL Optimized1/3(restart)
  CORDIC Square Root HDL Optimized1/2(validOut) -> validOut/1
  Data Type Conversion/1 -> absolute/1
  Add/1 -> CORDIC Square Root HDL Optimized1/1(u)
  CORDIC Square Root HDL Optimized1/1(y) -> Data Type Conversion/1
  inrepeat/1 -> t/1
  Constant1/1 -> HwModeRegister2/1, HwModeRegister5/1
  Multiply-Add1_out_dtc/1 -> Add/2
  Multiply-Add_out_dtc/1 -> Add/1
  t/1 -> HwModeRegister3/1, HwModeRegister4/1
  t/2 -> HwModeRegister/1, HwModeRegister1/1
  PipelineRegister/1 -> Multiply-Add1_out_dtc/1
  PipelineRegister1/1 -> Multiply-Add_out_dtc/1
  Multiply-Add1/1 -> PipelineRegister/1
  HwModeRegister/1 -> Multiply-Add1/1
  HwModeRegister1/1 -> Multiply-Add1/2
  HwModeRegister2/1 -> Multiply-Add1/3
  Multiply-Add/1 -> PipelineRegister1/1
  HwModeRegister3/1 -> Multiply-Add/1
  HwModeRegister4/1 -> Multiply-Add/2
  HwModeRegister5/1 -> Multiply-Add/3

== system gm_hdl_model_fixed/Subsystem1/Subsystem Reference/CORDIC Square Root HDL Optimized ==
  u : Inport  OutDataTypeStr=fixdt(1, 22, 20)  SampleTime=1e-08
  validIn : Inport  Port=2  OutDataTypeStr=boolean  SampleTime=1e-08
  restart : Inport  Port=3  OutDataTypeStr=boolean  SampleTime=1e-08
  Bit Shift Arithmetic : Subsystem
  Cast to Union of Types : Subsystem
  Data Type Conversion : DataTypeConversion  OutDataTypeStr=fixdt(1,22,20)
  Synchronous Subsystem : Subsystem
  y : Outport  SampleTime=1e-08
  validOut : Outport  Port=2  SampleTime=1e-08
  wires:
  u/1 -> Synchronous Subsystem/1(u), Cast to Union of Types/1(Xref)
  validIn/1 -> Synchronous Subsystem/2(validIn)
  restart/1 -> Synchronous Subsystem/3(restart)
  Data Type Conversion/1 -> y/1
  Synchronous Subsystem/1(dataOut) -> Cast to Union of Types/2(Cin)
  Synchronous Subsystem/2(eOut) -> Bit Shift Arithmetic/2(e)
  Synchronous Subsystem/3(isZero) -> Bit Shift Arithmetic/3(isZero)
  Synchronous Subsystem/4(validOut) -> validOut/1
  Cast to Union of Types/1(Cout) -> Bit Shift Arithmetic/1(u)
  Bit Shift Arithmetic/1(y) -> Data Type Conversion/1

== system gm_hdl_model_fixed/Subsystem1/Subsystem Reference/Real Divide HDL Optimized ==
  num : Inport  OutDataTypeStr=fixdt(1, 17, 14)  SampleTime=1e-08
  den : Inport  Port=2  OutDataTypeStr=fixdt(1, 17, 14)  SampleTime=5e-09
  validIn : Inport  Port=3  OutDataTypeStr=boolean  SampleTime=1e-08
  Delay1 : Delay  DelayLength=double(1)  InitialCondition=0  SampleTime=1e-08
  Delay17 : Delay  DelayLength=double(1)  InitialCondition=0  SampleTime=1e-08
  ForEach - Real Divide_instance1 : Subsystem
  Reshape to original size : Subsystem
  Verify divide sizes : Subsystem
  in1_repeat : dspsigops/Repeat  FactorSource=Dialog parameter  N=double(2)  Nmax=16  RateOptions=Allow multirate processing  ic=0  mode=Unused parameter value
  y = u(1) : Subsystem
  y : Outport  SampleTime=1e-08
  validOut : Outport  Port=2  SampleTime=1e-08
  wires:
  num/1 -> Reshape to original size/2(u), in1_repeat/1
  validIn/1 -> ForEach - Real Divide_instance1/3(validIn)
  ForEach - Real Divide_instance1/1(y) -> Reshape to original size/1(y)
  ForEach - Real Divide_instance1/2(validOut) -> y = u(1)/1(u)
  Delay1/1 -> validOut/1
  Delay17/1 -> y/1
  y = u(1)/1(y) -> Delay1/1
  Reshape to original size/1(z) -> Delay17/1
  den/1 -> Verify divide sizes/1(denominator)
  Verify divide sizes/1(den) -> ForEach - Real Divide_instance1/1(den)
  Verify divide sizes/2(num) -> ForEach - Real Divide_instance1/2(num)
  in1_repeat/1 -> Verify divide sizes/2(numerator)

== system gm_hdl_model_fixed/Subsystem1/Subsystem Reference/Sample and Hold ==
  In : Inport  OutDataTypeStr=fixdt(1, 16, 14)
  Trigger : TriggerPort  VariantControl=(inherit)  OutDataTypeStr=boolean
  " " : Outport  InitialOutput=0
  wires:
  In/1 -> " "/1

== system gm_hdl_model_fixed/Subsystem1/Subsystem Reference/Sample and Hold1 ==
  In : Inport  OutDataTypeStr=fixdt(1, 18, 10)
  Trigger : TriggerPort  VariantControl=(inherit)  OutDataTypeStr=boolean
  " " : Outport  InitialOutput=0
  wires:
  In/1 -> " "/1

== system gm_hdl_model_fixed/Subsystem1/Subsystem Reference/Sample and Hold2 ==
  In : Inport  OutDataTypeStr=fixdt(1, 22, 20)
  Trigger : TriggerPort  VariantControl=(inherit)  OutDataTypeStr=boolean
  " " : Outport  InitialOutput=0
  wires:
  In/1 -> " "/1

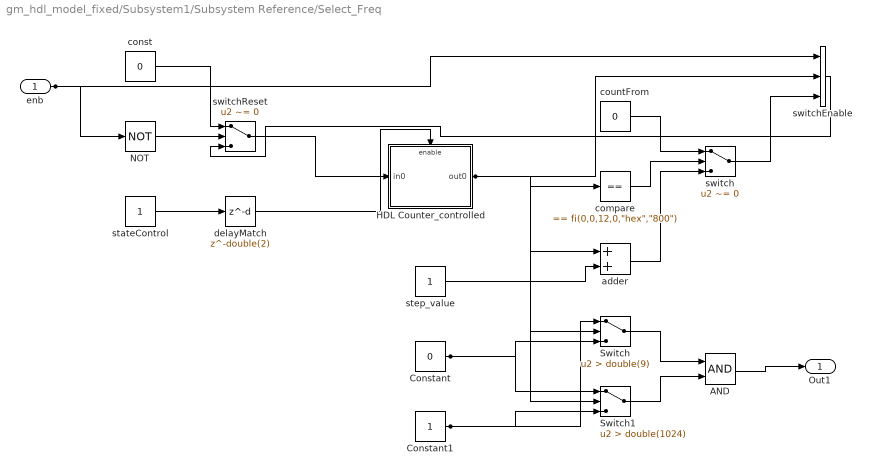
== system gm_hdl_model_fixed/Subsystem1/Subsystem Reference/Select_Freq ==
  enb : Inport  OutDataTypeStr=boolean  PortDimensions=1  SampleTime=1e-08
  AND : Logic  AllPortsSameDT=off  OutDataTypeStr=boolean  SampleTime=1e-08
  Constant : Constant  Value=0  OutDataTypeStr=boolean  SampleTime=1e-08
  Constant1 : Constant  OutDataTypeStr=boolean  SampleTime=1e-08
  HDL Counter_controlled : Subsystem
  NOT : Logic  Operator=NOT  Inputs=1  AllPortsSameDT=off  OutDataTypeStr=boolean  SampleTime=1e-08
  Switch : Switch  Criteria=u2 > Threshold  Threshold=double(9)  OutDataTypeStr=boolean  SampleTime=1e-08  SaturateOnIntegerOverflow=off  InputSameDT=off
  Switch1 : Switch  Criteria=u2 > Threshold  Threshold=double(1024)  OutDataTypeStr=boolean  SampleTime=1e-08  SaturateOnIntegerOverflow=off  InputSameDT=off
  adder : Sum  OutDataTypeStr=fixdt(0, 12, 0)  AccumDataTypeStr=fixdt(0, 12, 0)  SampleTime=1e-08
  compare : simulink/Logic and Bit Operations/Compare To Constant  relop===  const="fi(0,0,12,0,\"hex\",\"800\")"  OutDataTypeStr=boolean
  const : Constant  Value=0  VectorParams1D=off  OutDataTypeStr=fixdt(0, 12, 0)  SampleTime=1e-08
  countFrom : Constant  Value=0  VectorParams1D=off  OutDataTypeStr=fixdt(0, 12, 0)  SampleTime=1e-08
  delayMatch : Delay  DelayLength=double(2)  InitialCondition=0  SampleTime=1e-08
  stateControl : Constant  OutDataTypeStr=boolean  SampleTime=1e-08
  step_value : Constant  VectorParams1D=off  OutDataTypeStr=fixdt(0, 12, 0)  SampleTime=1e-08
  switch : Switch  Criteria=u2 ~= 0  Threshold=double(0)  OutDataTypeStr=fixdt(0, 12, 0)  SampleTime=1e-08  SaturateOnIntegerOverflow=off  InputSameDT=off
  switchEnable : MultiPortSwitch  DataPortOrder=Zero-based contiguous  Inputs=2  DiagnosticForDefault=None  zeroidx=on  OutDataTypeStr=fixdt(0, 12, 0)  SampleTime=1e-08  SaturateOnIntegerOverflow=off  InputSameDT=off
  switchReset : Switch  Criteria=u2 ~= 0  Threshold=double(0)  OutDataTypeStr=fixdt(0, 12, 0)  SampleTime=1e-08  SaturateOnIntegerOverflow=off  InputSameDT=off
  Out1 : Outport  OutDataTypeStr=boolean  SampleTime=1e-08
  wires:
  enb/1 -> NOT/1, switchEnable/1
  AND/1 -> Out1/1
  Constant/1 -> Switch/3, Switch1/1
  Switch1/1 -> AND/2
  Constant1/1 -> Switch/1, Switch1/3
  Switch/1 -> AND/1
  stateControl/1 -> delayMatch/1
  HDL Counter_controlled/1(out0) -> adder/1, compare/1, switchEnable/2, Switch/2, Switch1/2
  delayMatch/1 -> HDL Counter_controlled/Enable
  step_value/1 -> adder/2
  countFrom/1 -> switch/1
  const/1 -> switchReset/1
  NOT/1 -> switchReset/2
  switchReset/1 -> HDL Counter_controlled/1(in0)
  adder/1 -> switch/3
  compare/1 -> switch/2
  switch/1 -> switchEnable/3
  switchEnable/1 -> switchReset/3

== system gm_hdl_model_fixed/Subsystem1/myRMS/CORDIC Square Root HDL Optimized ==
  u : Inport  OutDataTypeStr=fixdt(0, 16, 7)  SampleTime=1e-08
  validIn : Inport  Port=2  OutDataTypeStr=boolean  SampleTime=1e-08
  restart : Inport  Port=3  OutDataTypeStr=boolean  SampleTime=1e-08
  Bit Shift Arithmetic : Subsystem
  Cast to Union of Types : Subsystem
  Data Type Conversion : DataTypeConversion  OutDataTypeStr=fixdt(0, 16, 7)  RndMeth=Nearest  SampleTime=1e-08  SaturateOnIntegerOverflow=off
  Synchronous Subsystem : Subsystem
  y : Outport  SampleTime=1e-08
  validOut : Outport  Port=2  SampleTime=1e-08
  wires:
  u/1 -> Synchronous Subsystem/1(u), Cast to Union of Types/1(Xref)
  validIn/1 -> Synchronous Subsystem/2(validIn)
  restart/1 -> Synchronous Subsystem/3(restart)
  Data Type Conversion/1 -> y/1
  Synchronous Subsystem/1(dataOut) -> Cast to Union of Types/2(Cin)
  Synchronous Subsystem/2(eOut) -> Bit Shift Arithmetic/2(e)
  Synchronous Subsystem/3(isZero) -> Bit Shift Arithmetic/3(isZero)
  Synchronous Subsystem/4(validOut) -> validOut/1
  Cast to Union of Types/1(Cout) -> Bit Shift Arithmetic/1(u)
  Bit Shift Arithmetic/1(y) -> Data Type Conversion/1

== system gm_hdl_model_fixed/Subsystem1/myRMS/Sample and Hold ==
  In : Inport  OutDataTypeStr=fixdt(0, 16, 7)
  Trigger : TriggerPort  VariantControl=(inherit)  OutDataTypeStr=boolean
  " " : Outport  InitialOutput=0
  wires:
  In/1 -> " "/1

== system gm_hdl_model_fixed/Subsystem1/Subsystem Reference/Absolute of Complex/CORDIC Square Root HDL Optimized1 ==
  u : Inport  OutDataTypeStr=fixdt(1, 24, 22)  SampleTime=5e-09
  validIn : Inport  Port=2  OutDataTypeStr=boolean  SampleTime=1e-08
  restart : Inport  Port=3  OutDataTypeStr=boolean  SampleTime=1e-08
  Bit Shift Arithmetic : Subsystem
  Cast to Union of Types : Subsystem
  Data Type Conversion : DataTypeConversion  OutDataTypeStr=fixdt(1,24,22)
  Synchronous Subsystem : Subsystem
  delayMatch : Delay  DelayLength=double(4)  InitialCondition=0  SampleTime=5e-09
  in1_repeat : dspsigops/Repeat  FactorSource=Dialog parameter  N=double(2)  Nmax=16  RateOptions=Allow multirate processing  ic=0  mode=Unused parameter value
  in2_repeat : dspsigops/Repeat  FactorSource=Dialog parameter  N=double(2)  Nmax=16  RateOptions=Allow multirate processing  ic=0  mode=Unused parameter value
  in3_repeat : dspsigops/Repeat  FactorSource=Dialog parameter  N=double(2)  Nmax=16  RateOptions=Allow multirate processing  ic=0  mode=Unused parameter value
  y : Outport  SampleTime=5e-09
  validOut : Outport  Port=2  SampleTime=1e-08
  wires:
  validIn/1 -> Synchronous Subsystem/2(validIn)
  restart/1 -> Synchronous Subsystem/3(restart)
  Synchronous Subsystem/1(dataOut) -> in1_repeat/1
  Synchronous Subsystem/2(eOut) -> in2_repeat/1
  Synchronous Subsystem/3(isZero) -> in3_repeat/1
  Synchronous Subsystem/4(validOut) -> validOut/1
  delayMatch/1 -> Cast to Union of Types/1(Xref)
  Data Type Conversion/1 -> y/1
  in1_repeat/1 -> Cast to Union of Types/2(Cin)
  in2_repeat/1 -> Bit Shift Arithmetic/2(e)
  in3_repeat/1 -> Bit Shift Arithmetic/3(isZero)
  u/1 -> delayMatch/1, Synchronous Subsystem/1(u)
  Cast to Union of Types/1(Cout) -> Bit Shift Arithmetic/1(u)
  Bit Shift Arithmetic/1(y) -> Data Type Conversion/1

== system gm_hdl_model_fixed/Subsystem1/Subsystem Reference/CORDIC Square Root HDL Optimized/Bit Shift Arithmetic ==
  u : Inport  OutDataTypeStr=fixdt(1, 22, 20)  PortDimensions=1  SampleTime=1e-08
  e : Inport  Port=2  OutDataTypeStr=int32  PortDimensions=1  SampleTime=1e-08
  isZero : Inport  Port=3  OutDataTypeStr=boolean  PortDimensions=1  SampleTime=1e-08
  embmathops_c6_sxviEMGenxpVSWTChSq0GHG_Bit_Shift_Arithmetic : MATLAB Function  TreatAsAtomicUnit=on
      settings: LibrarySourceBlock=embmathops/CORDIC Square Root HDL Optimized/Bit Shift Arithmetic
  y : Outport  SampleTime=1e-08  VectorParamsAs1DForOutWhenUnconnected=off
  wires:
  u/1 -> embmathops_c6_sxviEMGenxpVSWTChSq0GHG_Bit_Shift_Arithmetic/1(u)
  e/1 -> embmathops_c6_sxviEMGenxpVSWTChSq0GHG_Bit_Shift_Arithmetic/2(e)
  isZero/1 -> embmathops_c6_sxviEMGenxpVSWTChSq0GHG_Bit_Shift_Arithmetic/3(isZero)
  embmathops_c6_sxviEMGenxpVSWTChSq0GHG_Bit_Shift_Arithmetic/1(y) -> y/1

== system gm_hdl_model_fixed/Subsystem1/Subsystem Reference/CORDIC Square Root HDL Optimized/Cast to Union of Types ==
  Xref : Inport  OutDataTypeStr=fixdt(1, 22, 20)  SampleTime=1e-08
  Cin : Inport  Port=2  OutDataTypeStr=fixdt(1, 22, 20)  SampleTime=1e-08
  slutils_c1_sUkuwzpcxqKl25e4GzDa0OH_Cast_to_Union_of_Types : MATLAB Function
      settings: LibrarySourceBlock=slutils/Cast to Union of Types
  Cout : Outport  SampleTime=1e-08
  wires:
  Xref/1 -> slutils_c1_sUkuwzpcxqKl25e4GzDa0OH_Cast_to_Union_of_Types/1(Xref)
  Cin/1 -> slutils_c1_sUkuwzpcxqKl25e4GzDa0OH_Cast_to_Union_of_Types/2(Cin)
  slutils_c1_sUkuwzpcxqKl25e4GzDa0OH_Cast_to_Union_of_Types/1(Cout) -> Cout/1

== system gm_hdl_model_fixed/Subsystem1/Subsystem Reference/CORDIC Square Root HDL Optimized/Synchronous Subsystem ==
  u : Inport  OutDataTypeStr=fixdt(1, 22, 20)  PortDimensions=1  SampleTime=1e-08
  validIn : Inport  Port=2  OutDataTypeStr=boolean  PortDimensions=1  SampleTime=1e-08
  restart : Inport  Port=3  OutDataTypeStr=boolean  PortDimensions=1  SampleTime=1e-08
  StateControl : StateControl  StateControl=Synchronous
  cordicSquareRootHDL : Subsystem
  dataOut : Outport  SampleTime=1e-08  VectorParamsAs1DForOutWhenUnconnected=off
  eOut : Outport  Port=2  SampleTime=1e-08  VectorParamsAs1DForOutWhenUnconnected=off
  isZero : Outport  Port=3  SampleTime=1e-08  VectorParamsAs1DForOutWhenUnconnected=off
  validOut : Outport  Port=4  SampleTime=1e-08  VectorParamsAs1DForOutWhenUnconnected=off
  wires:
  u/1 -> cordicSquareRootHDL/1(u)
  validIn/1 -> cordicSquareRootHDL/2(validIn)
  restart/1 -> cordicSquareRootHDL/3(restart)
  cordicSquareRootHDL/1(dataOut) -> dataOut/1
  cordicSquareRootHDL/2(eOut) -> eOut/1
  cordicSquareRootHDL/3(isZero) -> isZero/1
  cordicSquareRootHDL/4(validOut) -> validOut/1
